simulink model "AC_Vfinal"  (R2024a)
settings: Solver=VariableStepAuto  StartTime=0.0  StopTime=sim_time  RelTol=1e-3
values from neighbouring files (symbols this model uses):
  a1 = 0.125    [AC_v_final.m]
  A1 = 2.83    [AC_v_final.m]
  a2 = 0.027    [AC_v_final.m]
  A2 = 0.55    [AC_v_final.m]
  Ao = 30    [AC_v_final.m]
  Cp_C = 1.147    [AC_v_final.m]
  Cp_E = 1.366    [AC_v_final.m]
  Cpa = 1.008    [AC_v_final.m]
  Cpe = 1.008    [AC_v_final.m]
  cpl = 1.166    [AC_v_final.m]
  cpr = 1.008    [AC_v_final.m]
  cpr1 = 1.436    [AC_v_final.m]
  cpr2 = 0.955    [AC_v_final.m]
  cpv = 0.906    [AC_v_final.m]
  D = 0.14    [AC_v_final.m]
  f1 = 0.281    [AC_v_final.m]
  f2 = 0.115    [AC_v_final.m]
  hfg = .2450    (= 0.245)    [AC_v_final.m]
  hr1 = .2335    (= 0.2335)    [AC_v_final.m]
  hr2 = .4288    (= 0.4288)    [AC_v_final.m]
  Kf = 1.1    [AC_v_final.m]
  Mf = 0.001    [AC_v_final.m]
  Mfl = 0.001    [AC_v_final.m]
  Mfv = 0.01    [AC_v_final.m]
  mr = 9000.50    (= 9000.5)    [AC_v_final.m]
  N = 1    [AC_v_final.m]
  n = 6    [AC_v_final.m]
  Nc = 11.50    (= 11.5)    [AC_v_final.m]
  nv = (0.3596+(1.1072*sp)-(0.4025*sp*sp)+(0.0001175*Nc)-(2.449*1.0000e-08*Nc*Nc))    (= 0.806835761198)    [AC_v_final.m]
  P = 1.2    [AC_v_final.m]
  Qps = 70    [AC_v_final.m]
  Qs = 50    [AC_v_final.m]
  sp1 = 10    [AC_v_final.m]
  Ta = 21    [AC_v_final.m]
  Tin = 40    [AC_v_final.m]
  Uo = 4    [AC_v_final.m]
  V = 0.115    [AC_v_final.m]
  v = 8    [AC_v_final.m]
  Vh1 = 0.004    [AC_v_final.m]
  Vh2 = 0.016    [AC_v_final.m]
  vs = 0.087    [AC_v_final.m]
  Wg = 0.009    [AC_v_final.m]
  Wm = 0.0113    [AC_v_final.m]
settings Model: Creator=aravi  LastModifiedBy=jshah
settings SolverCC: AlgebraicLoopSolver=TrustRegion
settings DataIOCC: SaveFormat=StructureWithTime  ReturnWorkspaceOutputs=off
settings DebuggingCC: UnconnectedInputMsg=warning  UnconnectedOutputMsg=warning  UnconnectedLineMsg=warning
settings ModelReferenceCC: EnableRefExpFcnMdlSchedulingChecks=on
settings RTWCC: GPUComputeCapability=3.5

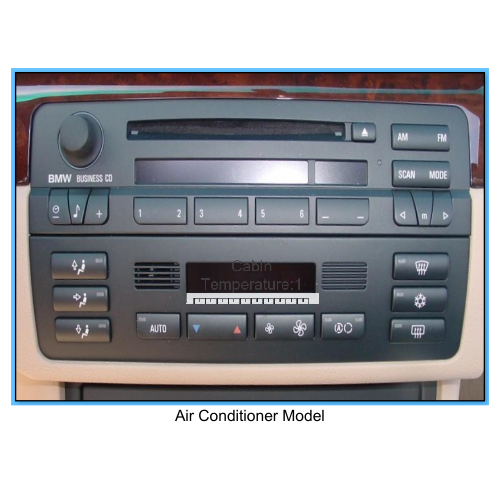
[thumbnail: Simulink's stored preview of the top-level diagram]
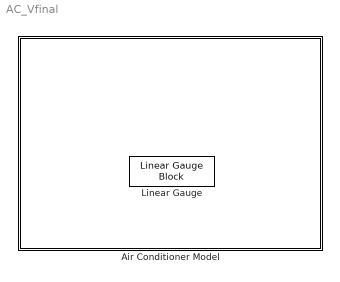
== system AC_Vfinal ==
  Air Conditioner Model : Subsystem
      mask Display: image('$imagefile'); % Use "Edit Image" on toolstrip to change.
  Linear Gauge : LinearGaugeBlock  ScaleMax=50  TickInterval=5

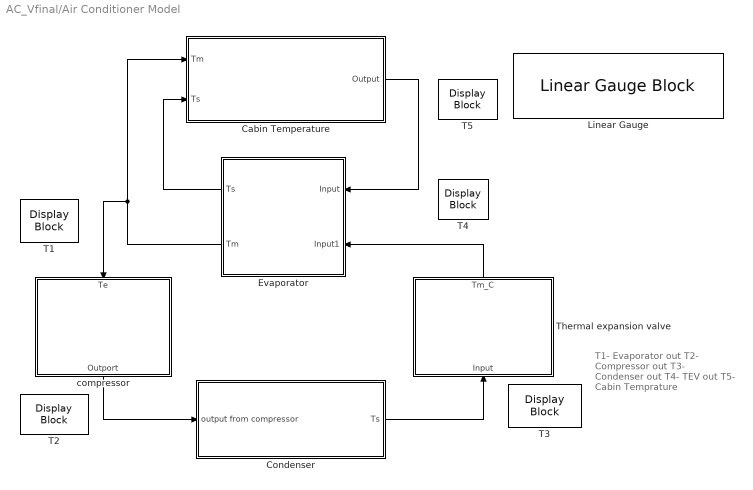
== system AC_Vfinal/Air Conditioner Model ==
  note: T1- Evaporator out
      | T2- Compressor out
      | T3- Condenser out
      | T4- TEV out
      | T5- Cabin Temprature
  Cabin Temperature : Subsystem
      mask Display: image('cabin.png');
  Condenser : Subsystem
      mask Display: image('condesner.png');
  Evaporator : Subsystem
      mask Display: image('evaporator.png');
  Linear Gauge : LinearGaugeBlock  ScaleMax=50  TickInterval=5
  T{1..5} (5 alike) : DisplayBlock  LabelPosition=Hide  Transparency=1
  Thermal expansion valve : Subsystem
      mask Display: image('EXV.jpg');
  compressor : Subsystem
      mask Display: image('compressor.jpg');
  wires:
  Evaporator/2(Tm) -> Cabin Temperature/1(Tm), compressor/1(Te)
  Condenser/1(Ts) -> Thermal expansion valve/1(Input)
  Cabin Temperature/1(Output) -> Evaporator/1(Input)
  compressor/1(Outport) -> Condenser/1(output from compressor)
  Thermal expansion valve/1(Tm_C) -> Evaporator/2(Input1)
  Evaporator/1(Ts) -> Cabin Temperature/2(Ts)

== system AC_Vfinal/Air Conditioner Model/Cabin Temperature ==
  Tm : Inport
  Ts : Inport  Port=2
  Temperature level : Subsystem
  Output : Outport
  wires:
  Tm/1 -> Temperature level/1(Tm)
  Temperature level/1(Output) -> Output/1
  Ts/1 -> Temperature level/2(Ts)

== system AC_Vfinal/Air Conditioner Model/Condenser ==
  output from compressor : Inport
  Mref : Subsystem
  Td block : Subsystem
  Tm block : Subsystem
  Ts block : Subsystem
  Tw block : Subsystem
  Ts : Outport
  wires:
  Ts block/2(Ts) -> Tw block/1(Ts)
  Tw block/1(Tw) -> Ts block/2(Tw), Td block/1(Tw)
  Td block/1(Td) -> Tw block/4(Td), Ts block/1(Td1)
  Ts block/1(Output to cabin Ts) -> Ts/1
  Tm block/1(Tm_C) -> Tw block/3(Tm), Td block/2(Tm)
  output from compressor/1 -> Tm block/1(Input)
  Mref/1(Out1) -> Tw block/2(Mref)

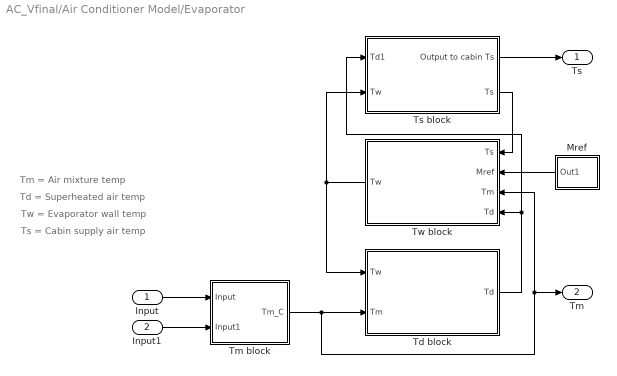
== system AC_Vfinal/Air Conditioner Model/Evaporator ==
  note: Ts = Cabin supply air temp
  note: Tw = Evaporator wall temp
  note: Td = Superheated air temp
  note: Tm = Air mixture temp
  Input : Inport
  Input1 : Inport  Port=2
  Mref : Subsystem
  Td block : Subsystem
  Tm block : Subsystem
  Ts block : Subsystem
  Tw block : Subsystem
  Ts : Outport
  Tm : Outport  Port=2
  wires:
  Ts block/2(Ts) -> Tw block/1(Ts)
  Td block/1(Td) -> Tw block/4(Td), Ts block/1(Td1)
  Tw block/1(Tw) -> Ts block/2(Tw), Td block/1(Tw)
  Ts block/1(Output to cabin Ts) -> Ts/1
  Tm block/1(Tm_C) -> Tm/1, Tw block/3(Tm), Td block/2(Tm)
  Input/1 -> Tm block/1(Input)
  Input1/1 -> Tm block/2(Input1)
  Mref/1(Out1) -> Tw block/2(Mref)

== system AC_Vfinal/Air Conditioner Model/Thermal expansion valve ==
  note: TinMfvcpv-ToutMflcpl = 0
  Input : Inport
  Gain1 : Gain  Gain=1/(Mfv*cpv)
  Gain4 : Gain  Gain=Mfl*cpl
  Scope2 : Scope
  Tm_C : Outport
  wires:
  Gain1/1 -> Scope2/1, Tm_C/1
  Input/1 -> Gain4/1
  Gain4/1 -> Gain1/1

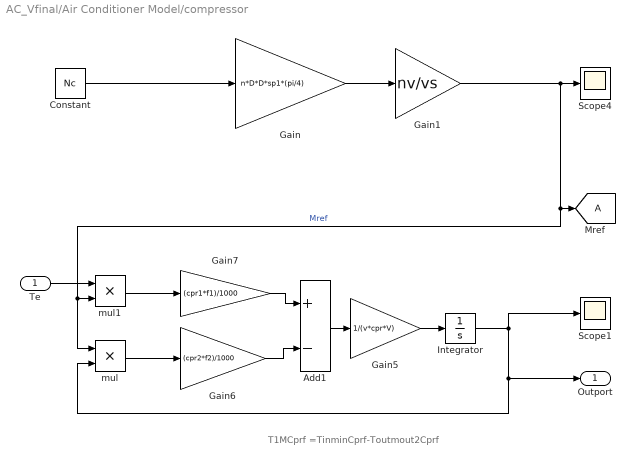
== system AC_Vfinal/Air Conditioner Model/compressor ==
  note: T1MCprf =TinminCprf-Toutmout2Cprf
  Te : Inport
  Add1 : Sum  Inputs=+-
  Constant : Constant  Value=Nc  VectorParams1D=off  SampleTime=-1
  Gain : Gain  Gain=n*D*D*sp1*(pi/4)
  Gain1 : Gain  Gain=nv/vs
  Gain5 : Gain  Gain=1/(v*cpr*V)
  Gain6 : Gain  Gain=(cpr2*f2)/1000
  Gain7 : Gain  Gain=(cpr1*f1)/1000
  Integrator : Integrator  InitialCondition=10
  Mref : Goto  TagVisibility=global
  Scope1 : Scope
  Scope4 : Scope
  mul : Product  Inputs=**
  mul1 : Product  Inputs=**
  Outport : Outport
  wires:
  Gain/1 -> Gain1/1
  Constant/1 -> Gain/1
  Integrator/1 -> Scope1/1, mul/2, Outport/1
  Add1/1 -> Gain5/1
  Gain6/1 -> Add1/2
  Gain7/1 -> Add1/1
  mul1/1 -> Gain7/1
  Gain5/1 -> Integrator/1
  Te/1 -> mul1/1
  Gain1/1 -> Scope4/1, Mref/1, mul/1, mul1/2  "Mref"
  mul/1 -> Gain6/1

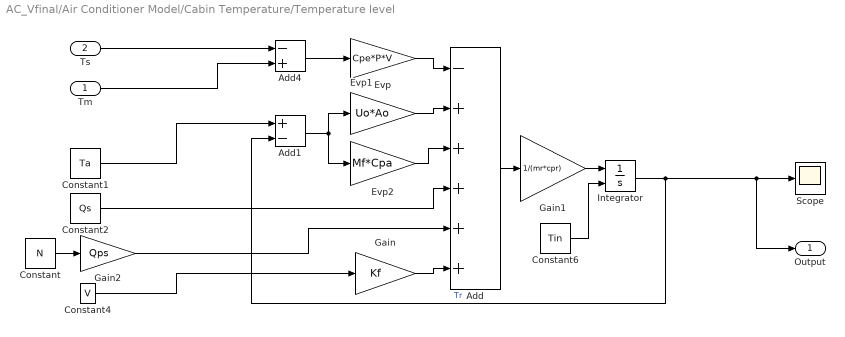
== system AC_Vfinal/Air Conditioner Model/Cabin Temperature/Temperature level ==
  Tm : Inport
  Ts : Inport  Port=2
  Add : Sum  Inputs=-+++++
  Add1 : Sum  Inputs=+-
  Add4 : Sum  Inputs=-+
  Constant : Constant  Value=N
  Constant1 : Constant  Value=Ta
  Constant2 : Constant  Value=Qs
  Constant4 : Constant  Value=V
  Constant6 : Constant  Value=Tin
  Evp : Gain  Gain=Cpe*P*V
  Evp1 : Gain  Gain=Uo*Ao
  Evp2 : Gain  Gain=Mf*Cpa
  Gain : Gain  Gain=Kf
  Gain1 : Gain  Gain=1/(mr*cpr)
  Gain2 : Gain  Gain=Qps
  Integrator : Integrator  InitialConditionSource=external
  Scope : Scope
  Output : Outport
  wires:
  Gain1/1 -> Integrator/1
  Constant2/1 -> Add/4
  Constant4/1 -> Gain/1
  Constant/1 -> Gain2/1
  Constant6/1 -> Integrator/2
  Evp1/1 -> Add/2
  Evp2/1 -> Add/3
  Gain/1 -> Add/6
  Evp/1 -> Add/1
  Add/1 -> Gain1/1
  Integrator/1 -> Add1/2, Output/1, Scope/1  "Tr"
  Add1/1 -> Evp2/1, Evp1/1
  Add4/1 -> Evp/1
  Constant1/1 -> Add1/1
  Tm/1 -> Add4/2
  Ts/1 -> Add4/1
  Gain2/1 -> Add/5

== system AC_Vfinal/Air Conditioner Model/Condenser/Mref ==
  From : From  TagVisibility=global
  Multiply : Gain  Gain=1/10
  Out1 : Outport
  wires:
  From/1 -> Multiply/1
  Multiply/1 -> Out1/1

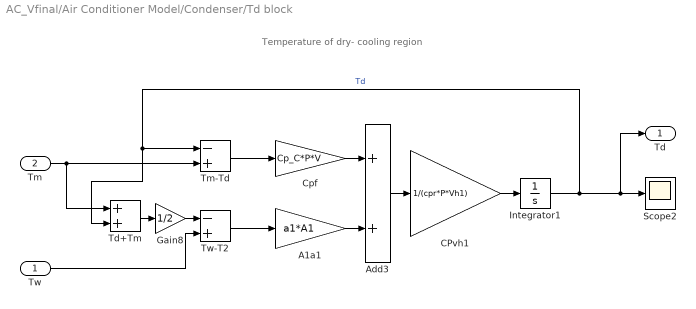
== system AC_Vfinal/Air Conditioner Model/Condenser/Td block ==
  note: Temperature of dry- cooling region
  Tw : Inport
  Tm : Inport  Port=2
  A1a1 : Gain  Gain=a1*A1
  Add3 : Sum
  CPvh1 : Gain  Gain=1/(cpr*P*Vh1)
  Cpf : Gain  Gain=Cp_C*P*V
  Gain8 : Gain  Gain=1/2
  Integrator1 : Integrator
  Scope2 : Scope
  Td+Tm : Sum
  Tm-Td : Sum  Inputs=-+
  Tw-T2 : Sum  Inputs=-+
  Td : Outport
  wires:
  Gain8/1 -> Tw-T2/1
  CPvh1/1 -> Integrator1/1
  Cpf/1 -> Add3/1
  Td+Tm/1 -> Gain8/1
  Tm-Td/1 -> Cpf/1
  Add3/1 -> CPvh1/1
  Integrator1/1 -> Td+Tm/2, Tm-Td/1, Td/1, Scope2/1  "Td"
  A1a1/1 -> Add3/2
  Tw-T2/1 -> A1a1/1
  Tw/1 -> Tw-T2/2
  Tm/1 -> Td+Tm/1, Tm-Td/2

== system AC_Vfinal/Air Conditioner Model/Condenser/Tm block ==
  note: ρfCpm Tm = mfCpaTa + (ρf − mf)CprTr
  Input : Inport
  Add1 : Sum
  Constant2 : Constant  Value=Ta
  Gain4 : Gain  Gain=Mf*Cpa
  Gain5 : Gain  Gain=(P*V-Mf)*cpr
  Gain6 : Gain  Gain=1/(P*V*Cp_C)
  Scope : Scope
  Tm_C : Outport
  wires:
  Gain5/1 -> Add1/2
  Add1/1 -> Gain6/1
  Constant2/1 -> Gain4/1
  Gain6/1 -> Scope/1, Tm_C/1
  Gain4/1 -> Add1/1
  Input/1 -> Gain5/1

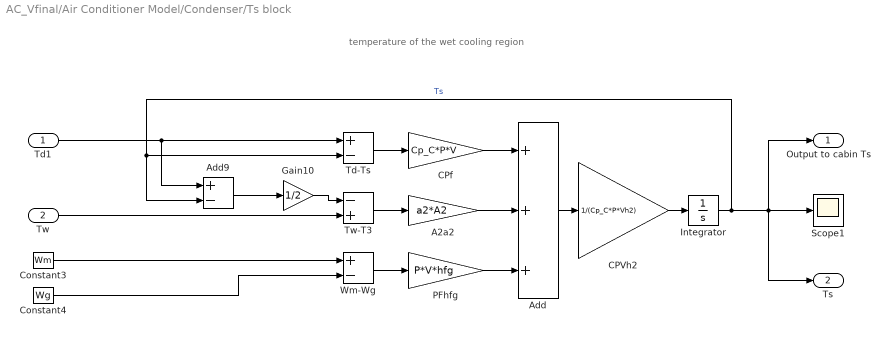
== system AC_Vfinal/Air Conditioner Model/Condenser/Ts block ==
  note: temperature of the wet cooling region
  Td1 : Inport
  Tw : Inport  Port=2
  A2a2 : Gain  Gain=a2*A2
  Add : Sum  Inputs=+++
  Add9 : Sum  Inputs=+-
  CPVh2 : Gain  Gain=1/(Cp_C*P*Vh2)
  CPf : Gain  Gain=Cp_C*P*V
  Constant3 : Constant  Value=Wm
  Constant4 : Constant  Value=Wg
  Gain10 : Gain  Gain=1/2
  Integrator : Integrator  InitialCondition=27
  PFhfg : Gain  Gain=P*V*hfg
  Scope1 : Scope
  Td-Ts : Sum  Inputs=+-
  Tw-T3 : Sum  Inputs=-+
  Wm-Wg : Sum  Inputs=+-
  Output to cabin Ts : Outport
  Ts : Outport  Port=2
  wires:
  Constant3/1 -> Wm-Wg/1
  CPVh2/1 -> Integrator/1
  Integrator/1 -> Add9/2, Td-Ts/2, Output to cabin Ts/1, Scope1/1, Ts/1  "Ts"
  Add/1 -> CPVh2/1
  Constant4/1 -> Wm-Wg/2
  CPf/1 -> Add/1
  Wm-Wg/1 -> PFhfg/1
  Gain10/1 -> Tw-T3/1
  Td1/1 -> Add9/1, Td-Ts/1
  Tw-T3/1 -> A2a2/1
  Tw/1 -> Tw-T3/2
  Add9/1 -> Gain10/1
  Td-Ts/1 -> CPf/1
  A2a2/1 -> Add/2
  PFhfg/1 -> Add/3

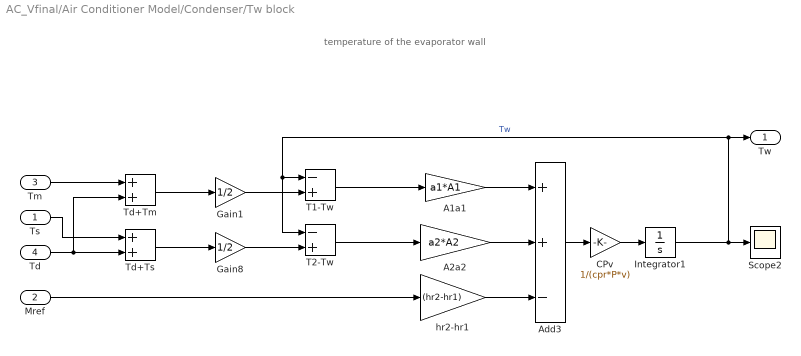
== system AC_Vfinal/Air Conditioner Model/Condenser/Tw block ==
  note: temperature of the evaporator wall
  Ts : Inport
  Mref : Inport  Port=2
  Tm : Inport  Port=3
  Td : Inport  Port=4
  A1a1 : Gain  Gain=a1*A1
  A2a2 : Gain  Gain=a2*A2
  Add3 : Sum  Inputs=++-
  CPv : Gain  Gain=1/(cpr*P*v)
  Gain1 : Gain  Gain=1/2
  Gain8 : Gain  Gain=1/2
  Integrator1 : Integrator  InitialCondition=28
  Scope2 : Scope
  T1-Tw : Sum  Inputs=-+
  T2-Tw : Sum  Inputs=-+
  Td+Tm : Sum
  Td+Ts : Sum
  hr2-hr1 : Gain  Gain=(hr2-hr1)
  Tw : Outport
  wires:
  T2-Tw/1 -> A2a2/1
  A2a2/1 -> Add3/2
  Integrator1/1 -> Scope2/1, T1-Tw/1, T2-Tw/1, Tw/1  "Tw"
  Add3/1 -> CPv/1
  T1-Tw/1 -> A1a1/1
  A1a1/1 -> Add3/1
  CPv/1 -> Integrator1/1
  Gain1/1 -> T1-Tw/2
  Td/1 -> Td+Tm/2, Td+Ts/2
  Gain8/1 -> T2-Tw/2
  Ts/1 -> Td+Ts/1
  Td+Tm/1 -> Gain1/1
  Td+Ts/1 -> Gain8/1
  hr2-hr1/1 -> Add3/3
  Tm/1 -> Td+Tm/1
  Mref/1 -> hr2-hr1/1

== system AC_Vfinal/Air Conditioner Model/Evaporator/Mref ==
  From : From  TagVisibility=global
  Gain : Gain  Gain=1/100
  Out1 : Outport
  wires:
  From/1 -> Gain/1
  Gain/1 -> Out1/1

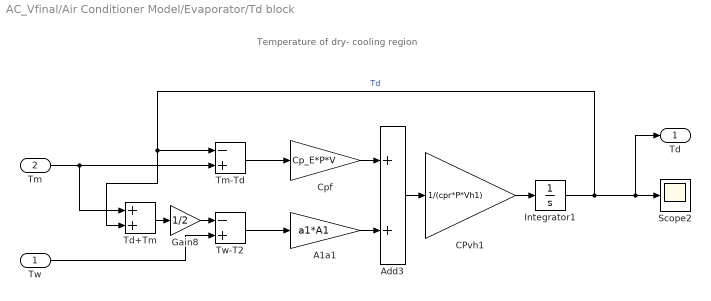
== system AC_Vfinal/Air Conditioner Model/Evaporator/Td block ==
  note: Temperature of dry- cooling region
  Tw : Inport
  Tm : Inport  Port=2
  A1a1 : Gain  Gain=a1*A1
  Add3 : Sum
  CPvh1 : Gain  Gain=1/(cpr*P*Vh1)
  Cpf : Gain  Gain=Cp_E*P*V
  Gain8 : Gain  Gain=1/2
  Integrator1 : Integrator  InitialCondition=27
  Scope2 : Scope
  Td+Tm : Sum
  Tm-Td : Sum  Inputs=-+
  Tw-T2 : Sum  Inputs=-+
  Td : Outport
  wires:
  Gain8/1 -> Tw-T2/1
  CPvh1/1 -> Integrator1/1
  Cpf/1 -> Add3/1
  Td+Tm/1 -> Gain8/1
  Tm-Td/1 -> Cpf/1
  Add3/1 -> CPvh1/1
  Integrator1/1 -> Td+Tm/2, Tm-Td/1, Td/1, Scope2/1  "Td"
  A1a1/1 -> Add3/2
  Tw-T2/1 -> A1a1/1
  Tw/1 -> Tw-T2/2
  Tm/1 -> Td+Tm/1, Tm-Td/2

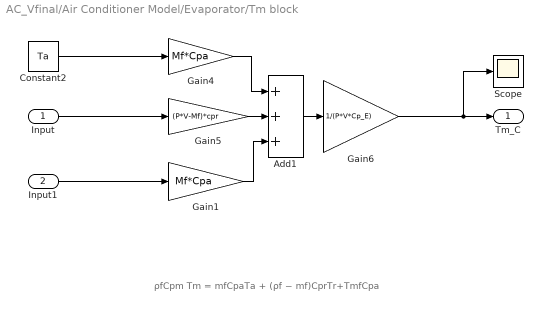
== system AC_Vfinal/Air Conditioner Model/Evaporator/Tm block ==
  note: ρfCpm Tm = mfCpaTa + (ρf − mf)CprTr+TmfCpa
  Input : Inport
  Input1 : Inport  Port=2
  Add1 : Sum  Inputs=+++
  Constant2 : Constant  Value=Ta
  Gain1 : Gain  Gain=Mf*Cpa
  Gain4 : Gain  Gain=Mf*Cpa
  Gain5 : Gain  Gain=(P*V-Mf)*cpr
  Gain6 : Gain  Gain=1/(P*V*Cp_E)
  Scope : Scope
  Tm_C : Outport
  wires:
  Gain5/1 -> Add1/2
  Add1/1 -> Gain6/1
  Input/1 -> Gain5/1
  Constant2/1 -> Gain4/1
  Gain6/1 -> Scope/1, Tm_C/1
  Gain4/1 -> Add1/1
  Input1/1 -> Gain1/1
  Gain1/1 -> Add1/3

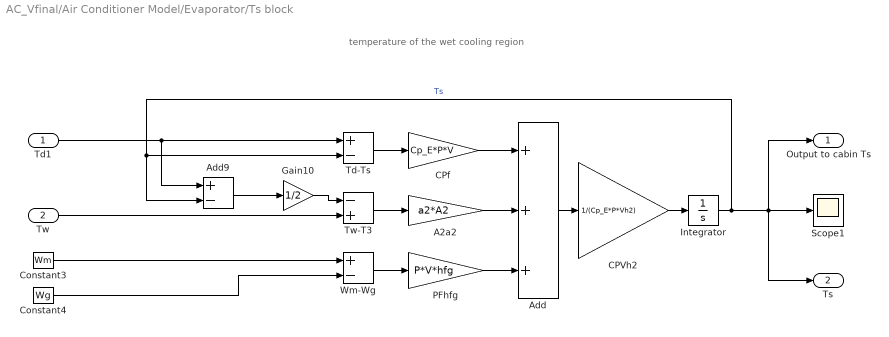
== system AC_Vfinal/Air Conditioner Model/Evaporator/Ts block ==
  note: temperature of the wet cooling region
  Td1 : Inport
  Tw : Inport  Port=2
  A2a2 : Gain  Gain=a2*A2
  Add : Sum  Inputs=+++
  Add9 : Sum  Inputs=+-
  CPVh2 : Gain  Gain=1/(Cp_E*P*Vh2)
  CPf : Gain  Gain=Cp_E*P*V
  Constant3 : Constant  Value=Wm
  Constant4 : Constant  Value=Wg
  Gain10 : Gain  Gain=1/2
  Integrator : Integrator  InitialCondition=27
  PFhfg : Gain  Gain=P*V*hfg
  Scope1 : Scope
  Td-Ts : Sum  Inputs=+-
  Tw-T3 : Sum  Inputs=-+
  Wm-Wg : Sum  Inputs=+-
  Output to cabin Ts : Outport
  Ts : Outport  Port=2
  wires:
  Constant3/1 -> Wm-Wg/1
  CPVh2/1 -> Integrator/1
  Integrator/1 -> Add9/2, Td-Ts/2, Output to cabin Ts/1, Scope1/1, Ts/1  "Ts"
  Add/1 -> CPVh2/1
  Constant4/1 -> Wm-Wg/2
  CPf/1 -> Add/1
  Wm-Wg/1 -> PFhfg/1
  Gain10/1 -> Tw-T3/1
  Td1/1 -> Add9/1, Td-Ts/1
  Tw-T3/1 -> A2a2/1
  Tw/1 -> Tw-T3/2
  Add9/1 -> Gain10/1
  Td-Ts/1 -> CPf/1
  A2a2/1 -> Add/2
  PFhfg/1 -> Add/3

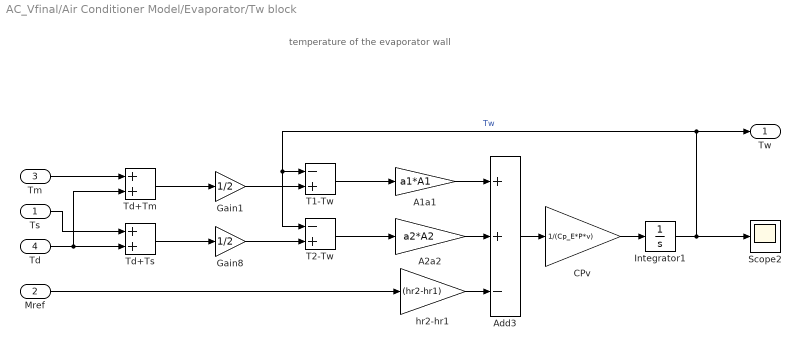
== system AC_Vfinal/Air Conditioner Model/Evaporator/Tw block ==
  note: temperature of the evaporator wall
  Ts : Inport
  Mref : Inport  Port=2
  Tm : Inport  Port=3
  Td : Inport  Port=4
  A1a1 : Gain  Gain=a1*A1
  A2a2 : Gain  Gain=a2*A2
  Add3 : Sum  Inputs=++-
  CPv : Gain  Gain=1/(Cp_E*P*v)
  Gain1 : Gain  Gain=1/2
  Gain8 : Gain  Gain=1/2
  Integrator1 : Integrator  InitialCondition=28
  Scope2 : Scope
  T1-Tw : Sum  Inputs=-+
  T2-Tw : Sum  Inputs=-+
  Td+Tm : Sum
  Td+Ts : Sum
  hr2-hr1 : Gain  Gain=(hr2-hr1)
  Tw : Outport
  wires:
  T2-Tw/1 -> A2a2/1
  A2a2/1 -> Add3/2
  Integrator1/1 -> Scope2/1, Tw/1, T1-Tw/1, T2-Tw/1  "Tw"
  Add3/1 -> CPv/1
  T1-Tw/1 -> A1a1/1
  A1a1/1 -> Add3/1
  CPv/1 -> Integrator1/1
  Gain1/1 -> T1-Tw/2
  Td/1 -> Td+Tm/2, Td+Ts/2
  Gain8/1 -> T2-Tw/2
  Ts/1 -> Td+Ts/1
  Td+Tm/1 -> Gain1/1
  Td+Ts/1 -> Gain8/1
  hr2-hr1/1 -> Add3/3
  Tm/1 -> Td+Tm/1
  Mref/1 -> hr2-hr1/1
